simulink model "aab_ut"  (Simulink 8.1)
settings: Solver=FixedStepDiscrete  StartTime=0.0  StopTime=Inf  FixedStep=0.005  RelTol=1e-3
PostLoadFcn:
  | , if any(exist('dsrtsu_mdlpostloadfcn', 'file') == [2, 3, 6]), try dsrtsu_mdlpostloadfcn('Execute', bdroot); catch fprintf('Error in PostLoadFcn (dsrtsu_mdlpostloadfcn) for model "%s":\n %s\n', bdroot, lasterr); end, end,
libraries: aab x1
settings Model: DSRTSU_INTERNAL_RTI_VER=450  DSRTSU_INTERNAL_RTI_TYPE=rti1401  RTICANMMDATA=struct('GeneralSetupData',struct('modelroot','D:\ELN150201_TAIWAN\trunk\AdasDragon\software\sw_development\arch\app\jud','generalsettings',struct('filesettings',struct('destfolder',struct('Name','RTICANMM_FILES','Check',1),'buildfolder',struct('Name','.','Check',1),'AbsDestfolder',struct('Name','D:\ELN150201_TAIWAN\trunk\AdasDragon\software\sw_development\arch\app\jud\RTICANMM_FILES'),'AbsBuildfolder',struct('Name','D:\ELN150201_TAIWAN\trunk\AdasDragon\software\sw_development\arch\app\jud'))),'options',struct('addpaths',1,'rmpaths',1,'addtrcexclusion',logical(1),'cannavigator',struct('checkmonitoring',0),'show_usrtrc',0,'use_usrtrc',0),'advanced',struct('options',[1 1 1 1 1 1 1 1 1 1 1 1 1 1 1 1 1 1 1 1 1 1 1 1 1 1 1 1 1 1 1 1 1 1 1 1 1 1 1 1 1 1 1 1 1 1 1 1 1 1 1 1 1 1 1 1 1 1 1 1 1 1 1 1 1 1 1 1 1 1 1 1 1 1 1 1 1 1 1 1 1 1 1 1 1 1 1 1 1 1 1 1 1 1 1 1 1 1 1 1]),'MPSetup',{{}},'modelname','aab_ut','block','aab_ut'))  DSRTSU_INTERNAL_RTIFPGA=40  Creator=AT015411  LastModifiedBy=AT015555  BufferReuse=off
settings DataIOCC: SignalLoggingSaveFormat=Dataset
settings OptimizationCC: BlockReduction=off  OptimizeBlockIOStorage=off  BufferReuse=off  ExpressionFolding=off  ExpressionDepthLimit=128  LocalBlockOutputs=off
settings DebuggingCC: FcnCallInpInsideContextMsg=EnableAllAsError
settings HardwareCC: ProdIntDivRoundTo=Zero  ProdEndianess=BigEndian  ProdHWDeviceType=Generic->Custom  TargetIntDivRoundTo=Zero  TargetEndianess=BigEndian  TargetHWDeviceType=Generic->Custom
settings RTWCC: SystemTargetFile=rti1005.tlc  MakeCommand=make_rti  TemplateMakefile=rti1005.tmf  Description=dSPACE DS1005 Hardware Platform  ProcessScript=rti1005_make_rtw_hook
settings STFCustomTargetCC: CodeReplacementLibrary=ANSI_C  ParMdlRefBuildCompliant=on  GeneratePreprocessorConditionals=Disable all  MatFileLogging=on  SystemTargetFile=rti1005.tlc
settings GRTTargetCC: CompOptLevelCompliant=off  ConcurrentExecutionCompliant=off  ExtModeMexFile=noextcomm
settings CustomProperty: DataType=RTWOptions_EnumType_C__Program Files (x86)_dSPACE RCPHIL 2014-B_MATLAB_RTI_RTI1401_TLC_rti1005_1InitialSimState  Value=RUN
settings EnumStrPairs: String=RUN

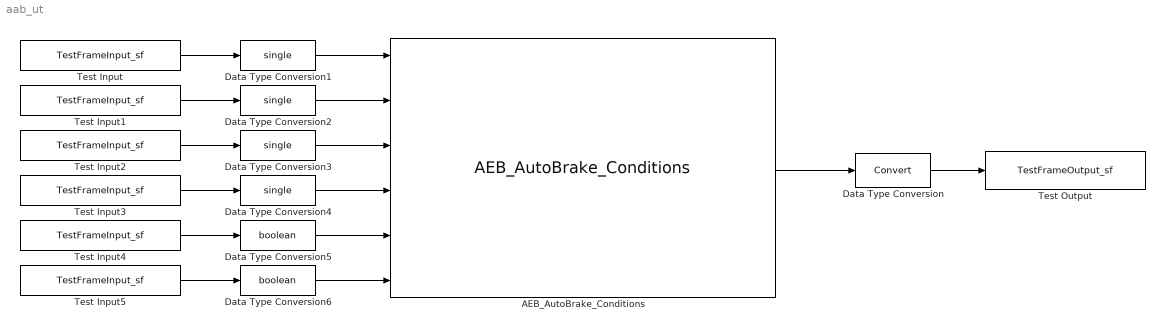
== system aab_ut ==
  AEB_AutoBrake_Conditions : aab/AEB_AutoBrake_Conditions
  Data Type Conversion : DataTypeConversion
  Data Type Conversion{1..4} (4 alike) : DataTypeConversion  OutDataTypeStr=single
  Data Type Conversion5 : DataTypeConversion  OutDataTypeStr=boolean
  Data Type Conversion6 : DataTypeConversion  OutDataTypeStr=boolean
  Test Input : S-Function  FunctionName=TestFrameInput_sf  Parameters=varname,sampletime  EnableBusSupport=off  mask(Test Input){varname=VJUD_AEBPoinToBrake_m, sampletime=0.005}
      mask prompts: varname "Name:"; sampletime "Sample Time:"
      mask help: Outputs the value of a Test Input variable from an Excel spreadsheet when used with the runsiltest script. Otherwise outputs 0.
      mask Display: fprintf('Test Input:\n%s',varname);
  Test Input1 : S-Function  FunctionName=TestFrameInput_sf  Parameters=varname,sampletime  EnableBusSupport=off  mask(Test Input){varname=VJUD_VRUPointToBrake_m, sampletime=0.005}
      mask prompts: varname "Name:"; sampletime "Sample Time:"
      mask help: Outputs the value of a Test Input variable from an Excel spreadsheet when used with the runsiltest script. Otherwise outputs 0.
      mask Display: fprintf('Test Input:\n%s',varname);
  Test Input2 : S-Function  FunctionName=TestFrameInput_sf  Parameters=varname,sampletime  EnableBusSupport=off  mask(Test Input){varname=VIFO_AEBVehClearance_m, sampletime=0.005}
      mask prompts: varname "Name:"; sampletime "Sample Time:"
      mask help: Outputs the value of a Test Input variable from an Excel spreadsheet when used with the runsiltest script. Otherwise outputs 0.
      mask Display: fprintf('Test Input:\n%s',varname);
  Test Input3 : S-Function  FunctionName=TestFrameInput_sf  Parameters=varname,sampletime  EnableBusSupport=off  mask(Test Input){varname=VIFO_VRUPedClearance_m, sampletime=0.005}
      mask prompts: varname "Name:"; sampletime "Sample Time:"
      mask help: Outputs the value of a Test Input variable from an Excel spreadsheet when used with the runsiltest script. Otherwise outputs 0.
      mask Display: fprintf('Test Input:\n%s',varname);
  Test Input4 : S-Function  FunctionName=TestFrameInput_sf  Parameters=varname,sampletime  EnableBusSupport=off  mask(Test Input){varname=VIFO_AEBTargetVehAssigned_flg, sampletime=0.005}
      mask prompts: varname "Name:"; sampletime "Sample Time:"
      mask help: Outputs the value of a Test Input variable from an Excel spreadsheet when used with the runsiltest script. Otherwise outputs 0.
      mask Display: fprintf('Test Input:\n%s',varname);
  Test Input5 : S-Function  FunctionName=TestFrameInput_sf  Parameters=varname,sampletime  EnableBusSupport=off  mask(Test Input){varname=VIFO_VRUTargetVehAssigned_flg, sampletime=0.005}
      mask prompts: varname "Name:"; sampletime "Sample Time:"
      mask help: Outputs the value of a Test Input variable from an Excel spreadsheet when used with the runsiltest script. Otherwise outputs 0.
      mask Display: fprintf('Test Input:\n%s',varname);
  Test Output : S-Function  FunctionName=TestFrameOutput_sf  Parameters=varname,sampletime  EnableBusSupport=off  mask(Test Output){varname=VJUD_AEBAutoBraking_flg, sampletime=-1}
      mask prompts: varname "Name:"; sampletime "Sample Time:"
      mask help: Samples the value of a Test Output variable from an Excel spreadsheet when used with the runsiltest script. Otherwise does nothing.
      mask Display: fprintf('Test Output:\n%s',varname);
  wires:
  AEB_AutoBrake_Conditions/1 -> Data Type Conversion/1
  Data Type Conversion/1 -> Test Output/1
  Test Input/1 -> Data Type Conversion1/1
  Data Type Conversion1/1 -> AEB_AutoBrake_Conditions/1
  Test Input1/1 -> Data Type Conversion2/1
  Data Type Conversion2/1 -> AEB_AutoBrake_Conditions/2
  Test Input2/1 -> Data Type Conversion3/1
  Data Type Conversion3/1 -> AEB_AutoBrake_Conditions/3
  Test Input3/1 -> Data Type Conversion4/1
  Data Type Conversion4/1 -> AEB_AutoBrake_Conditions/4
  Test Input4/1 -> Data Type Conversion5/1
  Data Type Conversion5/1 -> AEB_AutoBrake_Conditions/5
  Test Input5/1 -> Data Type Conversion6/1
  Data Type Conversion6/1 -> AEB_AutoBrake_Conditions/6
